simulink model "BrushlessDCmotorxt"  (Simulink 6.3)
settings: Solver=ode23t  StartTime=0  StopTime=0.2  FixedStep=Ts  MaxStep=1e-6  RelTol=1e-3  AbsTol=1e-3
PreLoadFcn:
  | assignin('base','Ts',[5e-6])
libraries: simulink x6, powerlib x5
Description:
  | This demonstration illustrates use of the BLDC in a closed-loop
  | speed and voltage control on a 1 kW, 3000 rpm industrial motor
settings Model: Creator=Olivier Tremblay  LastModifiedBy=Administrator  ExtModeAutoUpdateStatusClock=off  StrictBusMsg=None
settings DataIOCC: MaxDataPoints=10000000  SignalLoggingName=sigsOut
settings OptimizationCC: InlineInvariantSignals=on
settings DebuggingCC: SolverPrmCheckMsg=none  SigSpecEnsureSampleTimeMsg=none
settings HardwareCC: TargetUnknown=on

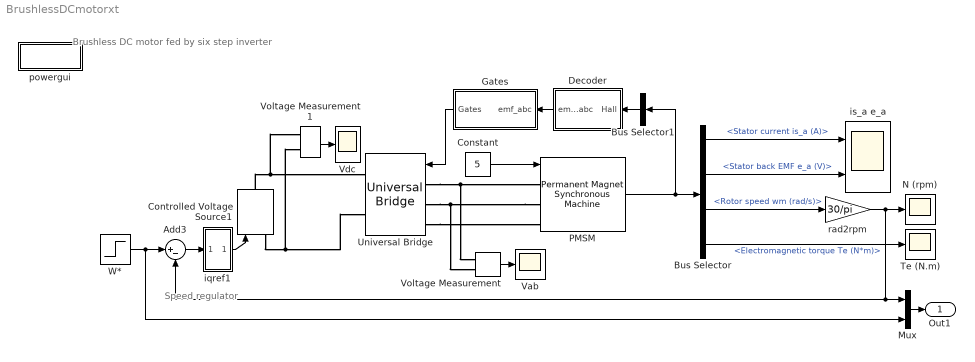
== system BrushlessDCmotorxt ==
  note: Brushless DC motor fed by six step inverter
  note: Speed
      | regulator
  Add3 : Sum  Inputs=|+-  OutScaling=2^-10
  Bus Selector : BusSelector  OutputSignals=Stator current is_a (A),Stator back EMF e_a (V),Rotor speed wm (rad/s),Electromagnetic torque Te (N*m)
  Bus Selector1 : BusSelector  Orientation=left  OutputSignals=Hall effect signal h_a,Hall effect signal h_b,Hall effect signal h_c  OutputAsBus=on
  Constant : Constant  Value=5
  Controlled Voltage Source1 : powerlib/Electrical Sources/Controlled Voltage Source  Orientation=up  Initialize=on  Amplitude=500  Phase=0  Frequency=0  Measurements=None
  Decoder : Subsystem  Orientation=left
  Gates : Subsystem  Orientation=left
  Mux : Mux  Inputs=2
  N (rpm) : Scope
      settings: TimeRange=0.2  YMin=0  YMax=3500  SaveName=N
  PMSM : powerlib/Machines/Permanent Magnet Synchronous Machine  FluxDistribution=Trapezoidal  MechanicalLoad=Torque Tm  PresetModel=No  ShowDetailedParameters=on  Resistance=2.8750  Inductance=8.5e-3  dqInductances=[8.5e-3, 8.5e-3]  Flux=0.175  Flat=120  Mechanical="[ 0.8e-3, 1e-3,  4 ]"
  Te (N.m) : Scope
      settings: TimeRange=0.2  YMin=0  YMax=3500  SaveName=N1
  Universal Bridge : powerlib/Power Electronics/Universal Bridge  Orientation=left  Arms=3  SnubberResistance=5000  SnubberCapacitance=1e-6  Device=MOSFET / Diodes  Ron=1e-3  Lon=0  ForwardVoltages="[  0  0  ]"  ForwardVoltage=0  GTOparameters=[ 10e-6 , 20e-6 ]  IGBTparameters=[ 1e-6 , 2e-6 ]  Measurements=None  converterType=Rectifier
  Vab : Scope
      settings: TimeRange=0.06  YMin=-10000  YMax=10000  SaveName=ScopeData4  DataFormat=Structure
  Vdc : Scope
      settings: TimeRange=0.2  YMin=0  YMax=500  SaveName=ScopeData3  DataFormat=Structure
  Voltage Measurement : powerlib/Measurements/Voltage Measurement  PhasorSimulation=off  OutputType=Complex  PSBequivalent=0
  Voltage Measurement1 : powerlib/Measurements/Voltage Measurement  PhasorSimulation=off  OutputType=Complex  PSBequivalent=0
  W* : Step  Time=.1  Before=2000  After=2800  SampleTime=0
  iqref1 : Subsystem  mask(PI Controller){@1=16.61, @2=.013, @3=[-500, 500]}
      mask prompts: @1 "Integral"; @2 "Proportional:"; @3 "Minimum and maximum outputs:"
      mask init:
      | I=@1;P=@2;sat=@3;min=sat(1);max=sat(2);
      mask Display: disp('PI')
  is_a e_a : Scope  NumInputPorts=2
      settings: TimeRange=0.2  YMin=-15~-250  YMax=20~250  SaveName=IE
  powergui : Subsystem  AncestorBlock=powerlib/powergui  mask(PSB option menu block){SimulationMode=Continuous, SampleTime=0, echomessages=off, x0status=blocks, Frange=[0:2:500], Ylog=off, Xlog=on, ShowGrid=off, save=off, variable=ZData, structure=, ZoomFFT=on, StartTime=0.0, cycles=1, DisplayStyle=1, fundamental=60, FreqAxis=off, MaxFrequency=1000, frequencyindice=1, frequencyindicesteady=1, RmsSteady=1, display=off, Ts=0, frequency=60, methode=off}
      mask prompts: SimulationMode "General parameter: Simulation Mode"; SampleTime "General parameter: Sample Time"; echomessages "General parameter: Echo  Messages"; x0status "Initial electrical states status"; Frange "Impedance tool: Frequency Range"; Ylog "Impedance tool: Log impedance"; Xlog "Impedance tool: log Frequency"; ShowGrid "Impedance tool: grid"; save "Impedance tool: Save Data To Workspace"; variable "Impedance tool: Variable Name"; structure "Structure Name (PSBFFTSCOPE)"; ZoomFFT "ZoomFFT (PSBFFTSCOPE)"; StartTime "Start Time (PSBFFTSCOPE)"; cycles "Cycles (PSBFFTSCOPE)"; DisplayStyle "Display style (PSBFFTSCOPE)"; fundamental "Fundamental (PSBFFTSCOPE)"; FreqAxis "Frequency Axis (PSBFFTSCOPE)"; MaxFrequency "Max Frequency (PSBFFTSCOPE)"; frequencyindice "Frequency indice  (PSBLOADFLOW)"; frequencyindicesteady "Frequency indice (STEADYSTATE)"; RmsSteady "RMS display (STEADYSTATE)"; display "Display Results"; Ts "Sample time (s):"; frequency "General parameter: phasor frequency"; methode "Phasor simulation"
      mask init:
      | powerlibroot = which('powersysdomain');
      | PSBroot = powerlibroot(1:end-16);
      | %
      | switch SimulationMode
      | 	case 1
      | 		message=sprintf('Continuous');
      | 	case 2
      |         message=sprintf('Discrete,\nTs = %.4g s.',SampleTime);
      | 	case 3
      | 		message=sprintf('Phasors');
      | end
      | if strcmp(bdroot,'powerlib')
      |   message='powergui';
      | end
      | power_initmask();
      settings: CopyFcn=powergui('Copy_Callback',gcb,0,[]);  DeleteFcn=powergui('Copy_Callback',gcb,1,[]);powergui('Close_Callback',gcb,[],[]);  ModelCloseFcn=powergui('Close_Callback',gcb,[],[]);  NameChangeFcn=handles = get_param(gcb,'UserData');if ~isempty(handles);delete(handles.powergui);end
      settings: PreSaveFcn=|
      | try
      | close(get_param(gcbh,'userdata'))
      | end
      settings: OpenFcn=|
      | if (power_openblockproxy ('secondary'))
      | powergui(gcb,'PM')
      | end;
      mask Help: web(psbhelp)
      mask StyleString: popup(Continuous|Discrete|Phasor),edit,checkbox,popup(blocks|steady|zero),edit,checkbox,checkbox,checkbox,checkbox,edit,edit,checkbox,edit,edit,edit,edit,checkbox,edit,edit,edit,edit,checkbox,edit,edit,checkbox
      mask Display: disp(message)
  rad2rpm : Gain  Gain=30/pi
  Out1 : Outport
  wires:
  W*/1 -> Add3/1, Mux/2
  iqref1/1(Out_1) -> Controlled Voltage Source1/1
  Add3/1 -> iqref1/1(In_1)
  Gates/1(Gates) -> Universal Bridge/1
  Decoder/1(emf_abc) -> Gates/1("emf_abc ")
  rad2rpm/1 -> N (rpm)/1, Add3/2, Mux/1
  Voltage Measurement/1 -> Vab/1
  Voltage Measurement1/1 -> Vdc/1
  Bus Selector/1 -> is_a e_a/1  "<Stator current is_a (A)>"
  PMSM/1 -> Bus Selector/1, Bus Selector1/1
  Bus Selector1/1 -> Decoder/1("Hall ")
  Bus Selector/2 -> is_a e_a/2  "<Stator back EMF e_a (V)>"
  Bus Selector/3 -> rad2rpm/1  "<Rotor speed wm (rad/s)>"
  Bus Selector/4 -> Te (N.m)/1  "<Electromagnetic torque Te (N*m)>"
  Constant/1 -> PMSM/1
  Mux/1 -> Out1/1
  connections:
  Universal Bridge/LConn1 -- PMSM/LConn1 -- Voltage Measurement/LConn1
  PMSM/LConn2 -- Universal Bridge/LConn2 -- Voltage Measurement/LConn2
  Universal Bridge/LConn3 -- PMSM/LConn3
  Controlled Voltage Source1/RConn1 -- Universal Bridge/RConn1 -- Voltage Measurement1/LConn1
  Controlled Voltage Source1/LConn1 -- Universal Bridge/RConn2 -- Voltage Measurement1/LConn2

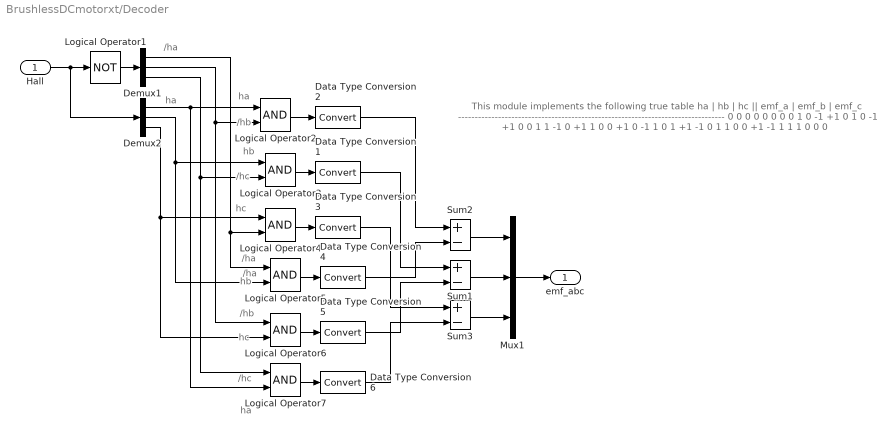
== system BrushlessDCmotorxt/Decoder ==
  note: /ha
  note: ha
  note: ha
  note: /hb
  note: hb
  note: /hc
  note: hc
  note: /ha
  note: /ha
  note: hb
  note: /hb
  note: hc
  note: /hc
  note: ha
  note: This module implements the following true table
      |
      |    ha   |   hb   |   hc   ||   emf_a   |   emf_b   |   emf_c
      |     --------------------------------------------------------------------------------
      | 0          0         0          0               0               0
      | 0          0         1          0               -1              +1
      | 0          1         0          -1              +1              0
      | 0          1         1          -1               0               +1
      | 1          0         0         +1               0               -1
      | 1          0         1         +1              -1                0
      | 1          1         0          0              +1               -1
      | 1          1         1          0               0                0
  "Hall " : Inport
  Data Type Conversion{1..6} (6 alike) : DataTypeConversion
  Demux1 : Demux  Outputs=3
  Demux2 : Demux  Outputs=3
  Logical Operator1 : Logic  Operator=NOT  AllPortsSameDT=off  OutDataTypeMode=Boolean
  Logical Operator{2..7} (6 alike) : Logic  AllPortsSameDT=off  OutDataTypeMode=Boolean
  Mux1 : Mux  Inputs=3
  Sum1 : Sum  Inputs=+-  OutDataTypeMode=double
  Sum2 : Sum  Inputs=+-  OutDataTypeMode=double
  Sum3 : Sum  Inputs=+-  OutDataTypeMode=double
  emf_abc : Outport
  wires:
  "Hall "/1 -> Logical Operator1/1, Demux2/1
  Logical Operator1/1 -> Demux1/1
  Demux2/3 -> Logical Operator4/1, Logical Operator6/2
  Demux2/2 -> Logical Operator5/2, Logical Operator3/1
  Demux2/1 -> Logical Operator2/1, Logical Operator7/2
  Demux1/3 -> Logical Operator3/2, Logical Operator7/1
  Demux1/2 -> Logical Operator2/2, Logical Operator6/1
  Demux1/1 -> Logical Operator4/2, Logical Operator5/1
  Logical Operator2/1 -> Data Type Conversion2/1
  Sum2/1 -> Mux1/1
  Sum1/1 -> Mux1/2
  Sum3/1 -> Mux1/3
  Mux1/1 -> emf_abc/1
  Logical Operator3/1 -> Data Type Conversion1/1
  Logical Operator4/1 -> Data Type Conversion3/1
  Logical Operator5/1 -> Data Type Conversion4/1
  Logical Operator6/1 -> Data Type Conversion5/1
  Logical Operator7/1 -> Data Type Conversion6/1
  Data Type Conversion2/1 -> Sum2/1
  Data Type Conversion4/1 -> Sum2/2
  Data Type Conversion1/1 -> Sum1/1
  Data Type Conversion5/1 -> Sum1/2
  Data Type Conversion3/1 -> Sum3/1
  Data Type Conversion6/1 -> Sum3/2

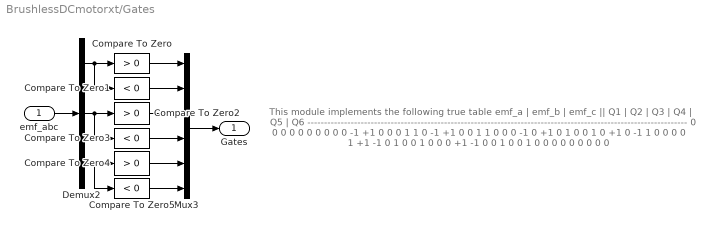
== system BrushlessDCmotorxt/Gates ==
  note: This module implements the following true table
      |
      |    emf_a   |   emf_b   |   emf_c   ||   Q1   |   Q2   |   Q3   |   Q4   |   Q5   |   Q6
      |     ------------------------------------------------------------------------------------------------------------------
      |       0              0                0            0          0          0           0        0        0
      |       0               -1              +1          0          0          0           1        1        0
      |     -1              +1                0          0          1          1           0        0        0
      |     -1               0               +1          0          1         0           0        1        0
      |    +1               0                -1          1          0          0           0        0        1
      |    +1              -1                0           1          0          0           1        0        0
      |      0              +1               -1           0          0          1           0        0        1
      |     0              0                0             0          0          0           0        0        0
  "emf_abc " : Inport
  Compare To Zero : simulink/Logic and Bit Operations/Compare To Zero  relop=>  LogicOutDataTypeMode=boolean  ZeroCross=off
  Compare To Zero1 : simulink/Logic and Bit Operations/Compare To Zero  relop=<  LogicOutDataTypeMode=boolean  ZeroCross=off
  Compare To Zero2 : simulink/Logic and Bit Operations/Compare To Zero  relop=>  LogicOutDataTypeMode=boolean  ZeroCross=off
  Compare To Zero3 : simulink/Logic and Bit Operations/Compare To Zero  relop=<  LogicOutDataTypeMode=boolean  ZeroCross=off
  Compare To Zero4 : simulink/Logic and Bit Operations/Compare To Zero  relop=>  LogicOutDataTypeMode=boolean  ZeroCross=off
  Compare To Zero5 : simulink/Logic and Bit Operations/Compare To Zero  relop=<  LogicOutDataTypeMode=boolean  ZeroCross=off
  Demux2 : Demux  Outputs=3
  Mux3 : Mux  Inputs=6
  Gates : Outport
  wires:
  "emf_abc "/1 -> Demux2/1
  Mux3/1 -> Gates/1
  Demux2/1 -> Compare To Zero/1, Compare To Zero1/1
  Compare To Zero/1 -> Mux3/1
  Compare To Zero1/1 -> Mux3/2
  Compare To Zero2/1 -> Mux3/3
  Compare To Zero3/1 -> Mux3/4
  Compare To Zero4/1 -> Mux3/5
  Compare To Zero5/1 -> Mux3/6
  Demux2/2 -> Compare To Zero2/1, Compare To Zero3/1
  Demux2/3 -> Compare To Zero4/1, Compare To Zero5/1

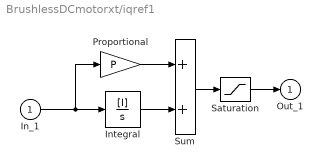
== system BrushlessDCmotorxt/iqref1 ==
  In_1 : Inport
  Integral : TransferFcn  Numerator=[I]  Denominator=[1 0]
  Proportional : Gain  Gain=P  SaturateOnIntegerOverflow=on
  Saturation : Saturate  UpperLimit=max  LowerLimit=min
  Sum : Sum  SaturateOnIntegerOverflow=on  InputSameDT=on
  Out_1 : Outport  InitialOutput=0
  wires:
  Saturation/1 -> Out_1/1
  Sum/1 -> Saturation/1
  Proportional/1 -> Sum/1
  In_1/1 -> Proportional/1, Integral/1
  Integral/1 -> Sum/2

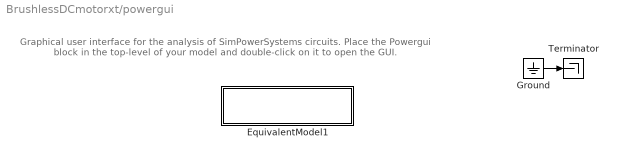
== system BrushlessDCmotorxt/powergui ==
  note: Graphical user interface for the analysis of  SimPowerSystems circuits.
      | Place the Powergui block in the top-level of your model and double-click
      | on it to open the GUI.
  EquivalentModel1 : Subsystem
      mask init:
      | SPS = get_param(gcbh,'UserData');
      | if isempty(SPS)
      |     A=0;
      |     B=0;
      |     C=0;
      |     D=0;
      |     x0=0;
      |     SwitchResistance=1;
      |     SwitchType=1;
      |     SwitchGateInitialValue=1;
      |     OutputsToResetToZero=1;
      | else
      | 	A=SPS.A;
      |     B=SPS.B;
      |     C=SPS.C;
      |     D=SPS.D;
      |     x0=SPS.x0;
      |     SwitchResistance=SPS.SwitchResistance;
      |     SwitchType=SPS.SwitchType;
      |     SwitchGateInitialValue=SPS.SwitchGateInitialValue;
      |     OutputsToResetToZero=SPS.YSwitchCurrent;
      | end
      mask Display:
      | color('blue')
      | disp('EQUIVALENT CIRCUIT')
  Ground : Ground
  Terminator : Terminator
  wires:
  Ground/1 -> Terminator/1

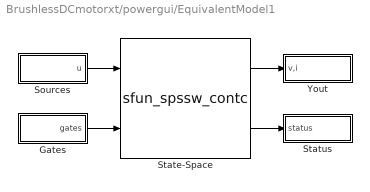
== system BrushlessDCmotorxt/powergui/EquivalentModel1 ==
  Gates : Subsystem
  Sources : Subsystem
  State-Space : S-Function  FunctionName=sfun_spssw_contc  Parameters=A, B, C, D, x0, SwitchResistance ,SwitchType, SwitchGateInitialValue, OutputsToResetToZero
  Status : Subsystem
  Yout : Subsystem
  wires:
  State-Space/1 -> Yout/1(v,i)
  State-Space/2 -> Status/1(status)
  Sources/1(u) -> State-Space/1
  Gates/1(gates) -> State-Space/2

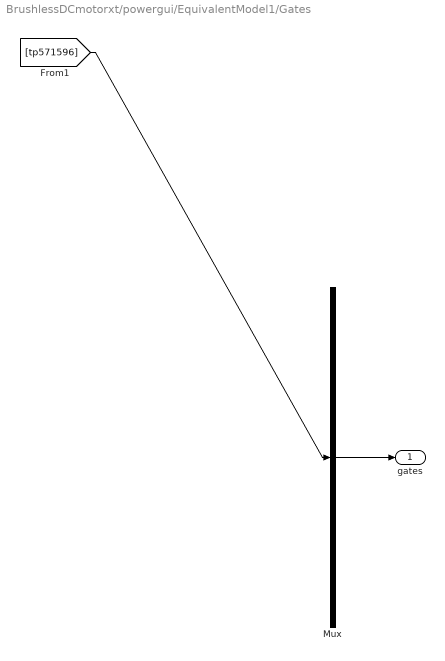
== system BrushlessDCmotorxt/powergui/EquivalentModel1/Gates ==
  Mux : Mux  Inputs=1
  gates : Outport
  wires:
  Mux/1 -> gates/1
  [tp571596] -> Mux/1

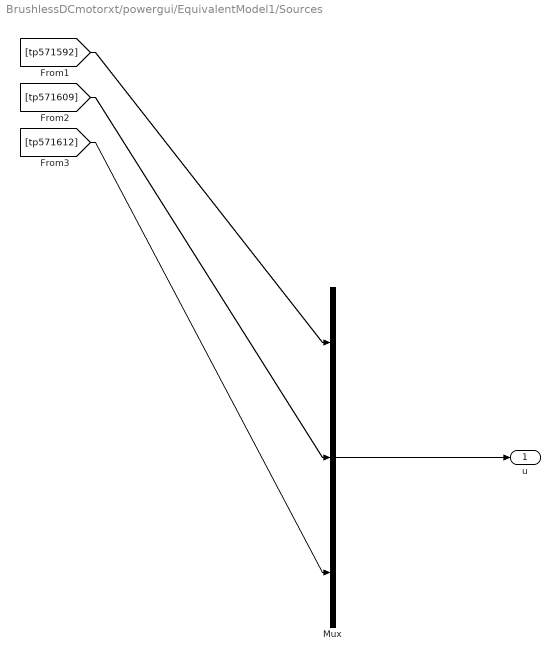
== system BrushlessDCmotorxt/powergui/EquivalentModel1/Sources ==
  Mux : Mux  Inputs=[6 2 1]
  u : Outport
  wires:
  Mux/1 -> u/1
  [tp571592] -> Mux/1
  [tp571609] -> Mux/2
  [tp571612] -> Mux/3

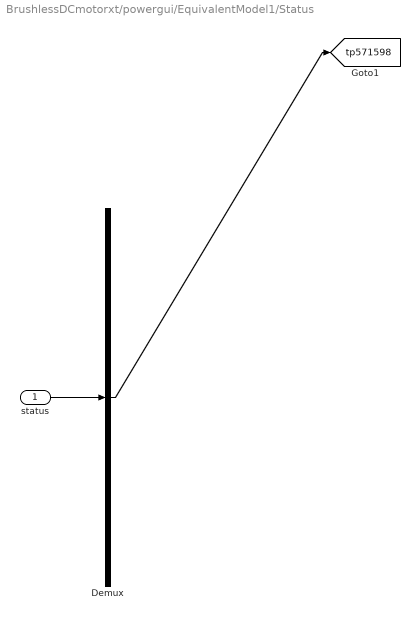
== system BrushlessDCmotorxt/powergui/EquivalentModel1/Status ==
  status : Inport
  Demux : Demux  Outputs=1
  tag scope: tp571598=global
  wires:
  status/1 -> Demux/1
  Demux/1 -> [tp571598]

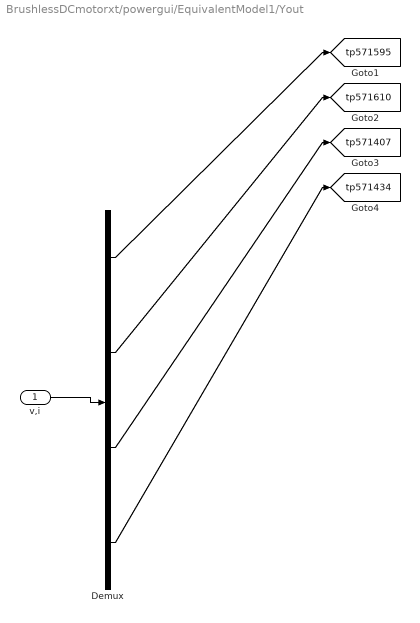
== system BrushlessDCmotorxt/powergui/EquivalentModel1/Yout ==
  v,i : Inport
  Demux : Demux  Outputs=[6 2 1 1]
  tag scope: tp571407=global, tp571434=global, tp571595=global, tp571610=global
  wires:
  v,i/1 -> Demux/1
  Demux/1 -> [tp571595]
  Demux/2 -> [tp571610]
  Demux/3 -> [tp571407]
  Demux/4 -> [tp571434]
